simulink model "lanechanging"  (R2021b)
settings: Solver=VariableStepAuto  StartTime=0.0  StopTime=t  RelTol=1e-3
values from neighbouring files (symbols this model uses):
  kd = 470    [longitudinal.m]
  kp = 2000    [longitudinal.m]
libraries: simulink_extras x6
settings Model: Creator=Dikshita Kothari  LastModifiedBy=Dikshita Kothari

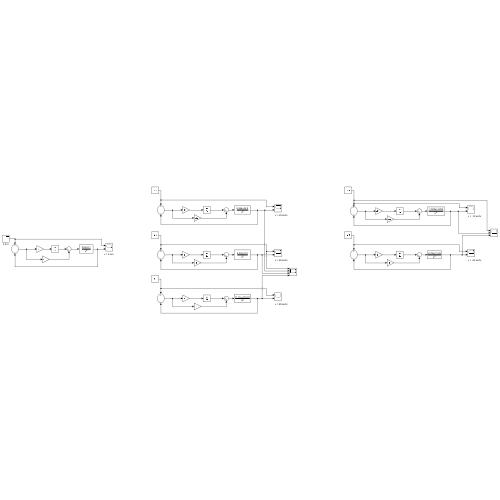
[thumbnail: Simulink's stored preview of the top-level diagram]
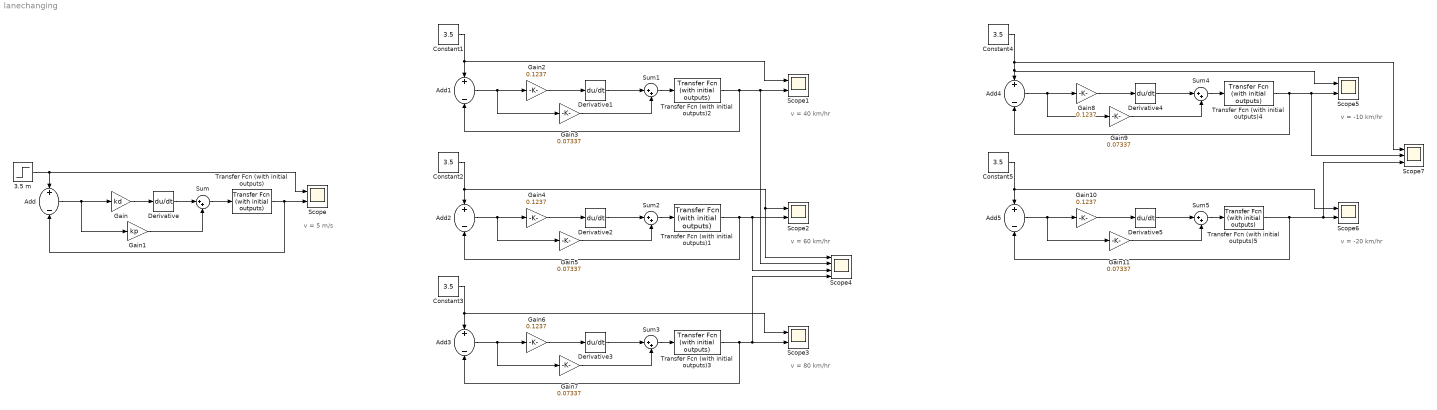
== system lanechanging ==
  note: v = 5 m/s
  note: v = 40 km/hr
  note: v = 60 km/hr
  note: v = 80 km/hr
  note: v = -10 km/hr
  note: v = -20 km/hr
  3.5 m : Step  Time=0  After=3.5  SampleTime=0
  Add{,1..5} (6 alike) : Sum  Inputs=+-
  Constant{1..5} (5 alike) : Constant  Value=3.5
  Derivative{,1..5} (6 alike) : Derivative
  Gain : Gain  Gain=kd
  Gain1 : Gain  Gain=kp
  Gain{2,4,6,8,10} (5 alike) : Gain  Gain=0.1237
  Gain{3,5,7,9,11} (5 alike) : Gain  Gain=0.07337
  Scope{,1..3,5..6} (6 alike) : Scope  NumInputPorts=2
  Scope4 : Scope  NumInputPorts=4
  Scope7 : Scope  NumInputPorts=3
  Sum{,1..5} (6 alike) : Sum  Inputs=|++
  Transfer Fcn (with initial outputs) : simulink_extras/Additional Linear/Transfer Fcn (with initial outputs)  N=[0.5 9.1]  D=[1 0 0]  Y0=0  U0=0
  Transfer Fcn (with initial outputs)1 : simulink_extras/Additional Linear/Transfer Fcn (with initial outputs)  N=[8.33 101]  D=[1 0 0]  Y0=0  U0=0
  Transfer Fcn (with initial outputs)2 : simulink_extras/Additional Linear/Transfer Fcn (with initial outputs)  N=[5.56 44.9]  D=[1 0 0]  Y0=0  U0=0
  Transfer Fcn (with initial outputs)3 : simulink_extras/Additional Linear/Transfer Fcn (with initial outputs)  N=[11.11 179.57]  D=[1 0 0]  Y0=0  U0=0
  Transfer Fcn (with initial outputs)4 : simulink_extras/Additional Linear/Transfer Fcn (with initial outputs)  N=[-1.389 2.805]  D=[1 0 0]  Y0=0  U0=0
  Transfer Fcn (with initial outputs)5 : simulink_extras/Additional Linear/Transfer Fcn (with initial outputs)  N=[-2.78 11.22]  D=[1 0 0]  Y0=0  U0=0
  wires:
  Transfer Fcn (with initial outputs)/1 -> Scope/2, Add/2
  Add/1 -> Gain/1, Gain1/1
  3.5 m/1 -> Scope/1, Add/1
  Gain/1 -> Derivative/1
  Sum/1 -> Transfer Fcn (with initial outputs)/1
  Derivative/1 -> Sum/1
  Gain1/1 -> Sum/2
  Add1/1 -> Gain2/1, Gain3/1
  Gain2/1 -> Derivative1/1
  Derivative1/1 -> Sum1/1
  Transfer Fcn (with initial outputs)2/1 -> Add1/2, Scope4/2, Scope1/2
  Constant1/1 -> Scope1/1, Add1/1
  Sum1/1 -> Transfer Fcn (with initial outputs)2/1
  Gain3/1 -> Sum1/2
  Transfer Fcn (with initial outputs)1/1 -> Add2/2, Scope2/2, Scope4/3
  Add2/1 -> Gain4/1, Gain5/1
  Derivative2/1 -> Sum2/1
  Gain5/1 -> Sum2/2
  Constant2/1 -> Scope2/1, Scope4/1, Add2/1
  Gain4/1 -> Derivative2/1
  Sum2/1 -> Transfer Fcn (with initial outputs)1/1
  Transfer Fcn (with initial outputs)3/1 -> Add3/2, Scope3/2, Scope4/4
  Add3/1 -> Gain6/1, Gain7/1
  Derivative3/1 -> Sum3/1
  Gain7/1 -> Sum3/2
  Constant3/1 -> Scope3/1, Add3/1
  Gain6/1 -> Derivative3/1
  Sum3/1 -> Transfer Fcn (with initial outputs)3/1
  Add4/1 -> Gain8/1, Gain9/1
  Gain8/1 -> Derivative4/1
  Derivative4/1 -> Sum4/1
  Transfer Fcn (with initial outputs)4/1 -> Add4/2, Scope7/2, Scope5/2
  Constant4/1 -> Scope7/1, Scope5/1, Add4/1
  Sum4/1 -> Transfer Fcn (with initial outputs)4/1
  Gain9/1 -> Sum4/2
  Add5/1 -> Gain10/1, Gain11/1
  Gain10/1 -> Derivative5/1
  Derivative5/1 -> Sum5/1
  Transfer Fcn (with initial outputs)5/1 -> Add5/2, Scope7/3, Scope6/2
  Constant5/1 -> Scope6/1, Add5/1
  Sum5/1 -> Transfer Fcn (with initial outputs)5/1
  Gain11/1 -> Sum5/2
